simulink model "Problem3_SinglePhase_Inverter"  (R2025b)
settings: Solver=ode23t  StartTime=0.0  StopTime=0.1  MaxStep=1e-5  RelTol=1e-3
settings Model: Creator=Rashid  LastModifiedBy=Rashid

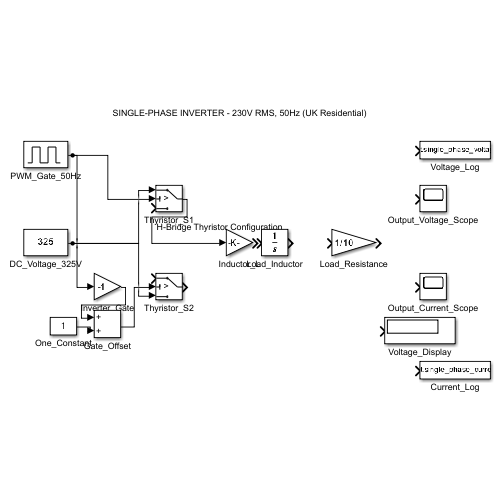
[thumbnail: Simulink's stored preview of the top-level diagram]
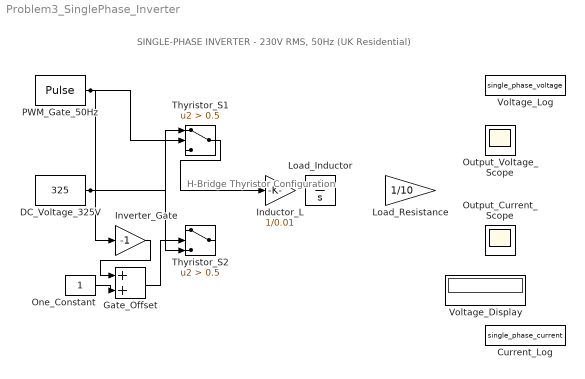
== system Problem3_SinglePhase_Inverter ==
  note: SINGLE-PHASE INVERTER - 230V RMS, 50Hz (UK Residential)
  note: H-Bridge Thyristor Configuration
  Current_Log : ToWorkspace  VariableName=single_phase_current  SaveFormat=Timeseries  SampleTime=-1
  DC_Voltage_325V : Constant  Value=325
  Gate_Offset : Sum
  Inductor_L : Gain  Gain=1/0.01
  Inverter_Gate : Gain  Gain=-1
  Load_Inductor : Integrator
  Load_Resistance : Gain  Gain=1/10
  One_Constant : Constant
  Output_Current_Scope : Scope
  Output_Voltage_Scope : Scope
  PWM_Gate_50Hz : DiscretePulseGenerator  PulseType=Time based  Period=0.02  PulseWidth=50
  Thyristor_S1 : Switch  Criteria=u2 > Threshold  Threshold=0.5  SaturateOnIntegerOverflow=off  InputSameDT=off
  Thyristor_S2 : Switch  Criteria=u2 > Threshold  Threshold=0.5  SaturateOnIntegerOverflow=off  InputSameDT=off
  Voltage_Display : Display
  Voltage_Log : ToWorkspace  VariableName=single_phase_voltage  SaveFormat=Timeseries  SampleTime=-1
  wires:
  PWM_Gate_50Hz/1 -> Thyristor_S1/2, Inverter_Gate/1
  Inverter_Gate/1 -> Gate_Offset/1
  One_Constant/1 -> Gate_Offset/2
  Gate_Offset/1 -> Thyristor_S2/2
  DC_Voltage_325V/1 -> Thyristor_S1/1, Thyristor_S2/3
  Thyristor_S1/1 -> Inductor_L/1
